simulink model "float_sch_PTSD"  (R2020a)
settings: Solver=VariableStepAuto  StartTime=0  StopTime=5  RelTol=1e-3
values from neighbouring files (symbols this model uses):
  buffer_rec = 30    [float_sch_run_PTSD.m]
  diff_th = [20:1.25:100]    [float_sch_run_PTSD.m]
  fs = 30000    [float_sch_run_LocalMaxima_AdaptiveThreshold.m]    (also in float_sch_run_LocalMaxima_HardThreshold.m; float_sch_run_PTSD.m; float_sch_run_Sample_AdaptiveThreshold.m; float_sch_run_Sample_HardThreshold.m)
  PLP = 22    [float_sch_run_PTSD.m]
  refractory = 10^-3    (= 0.001)    [float_sch_run_LocalMaxima_AdaptiveThreshold.m]    (also in float_sch_run_LocalMaxima_HardThreshold.m; float_sch_run_PTSD.m; float_sch_run_Sample_AdaptiveThreshold.m; float_sch_run_Sample_HardThreshold.m)
libraries: simulink x6, dsparch4 x2, dspstat3 x2, dspswit3 x1, hdlsllib x1
settings Model: Creator=sbuccelli  LastModifiedBy=diflo

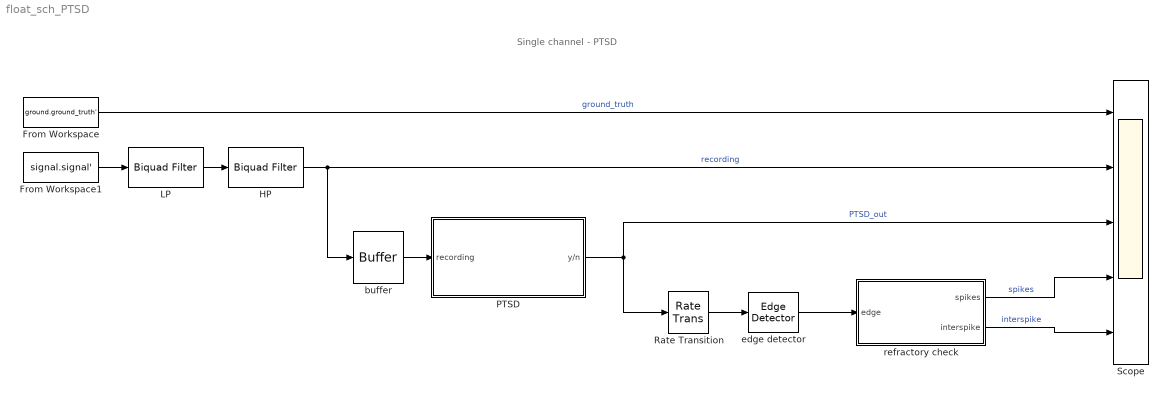
== system float_sch_PTSD ==
  note: Single channel - PTSD
  From Workspace : FromWorkspace  VariableName=ground.ground_truth'  SampleTime=1/fs
  From Workspace1 : FromWorkspace  VariableName=signal.signal'  SampleTime=1/fs
  HP : dsparch4/Biquad Filter  Tag=BlockMethodSubSystem  FilterSource=Dialog parameters  CoeffSource=Specify via dialog  FilterObject=BQF  IIRFiltStruct=Direct form II  BiQuadCoeffs=[1 -2 1 1 -1.93529438685999167 0.93912079880642374;1 -1 0 1 -0.939062505817492399 0]  ScaleValues=[0.968603796416603768;0.969531252908746199;1]  IC=0  ICnum=0  ICden=0  a0Flag=Warning  optimizeScaleValues=on  ScaleValueMode=Specify via input port (g)  roundingMode=Floor  overflowMode=off  scaleValueFracLength=14  denProdOutputFracLength=30  denAccumFracLength=30  secondMemoryFracLength=15
  LP : dsparch4/Biquad Filter  Tag=BlockMethodSubSystem  FilterSource=Dialog parameters  CoeffSource=Specify via dialog  FilterObject=BQF  IIRFiltStruct=Direct form II  BiQuadCoeffs=[1 1 0 1 -0.509525449494428795 0]  ScaleValues=[0.245237275252785547;1]  IC=0  ICnum=0  ICden=0  a0Flag=Warning  optimizeScaleValues=on  ScaleValueMode=Specify via input port (g)  roundingMode=Floor  overflowMode=off  scaleValueFracLength=14  denProdOutputFracLength=30  denAccumFracLength=30  secondMemoryFracLength=15
  PTSD : Subsystem
  Rate Transition : RateTransition  OutPortSampleTime=1/fs
  Scope : Scope  NumInputPorts=5
  buffer : Buffer  N=buffer_rec  V=buffer_overlap  OutputFrames=off
  edge detector : dspswit3/Edge Detector  InputProcessing=Columns as channels (frame based)
      settings: SourceProductBaseCode=DS
  refractory check : Subsystem
  wires:
  From Workspace/1 -> Scope/1  "ground_truth"
  buffer/1 -> PTSD/1(recording)
  From Workspace1/1 -> LP/1
  Rate Transition/1 -> edge detector/1
  PTSD/1(y/n) -> Scope/3, Rate Transition/1  "PTSD_out"
  refractory check/1(" spikes") -> Scope/4  "spikes"
  refractory check/2(interspike) -> Scope/5  "interspike"
  edge detector/1 -> refractory check/1(" edge  ")
  HP/1 -> Scope/2, buffer/1  "recording"
  LP/1 -> HP/1

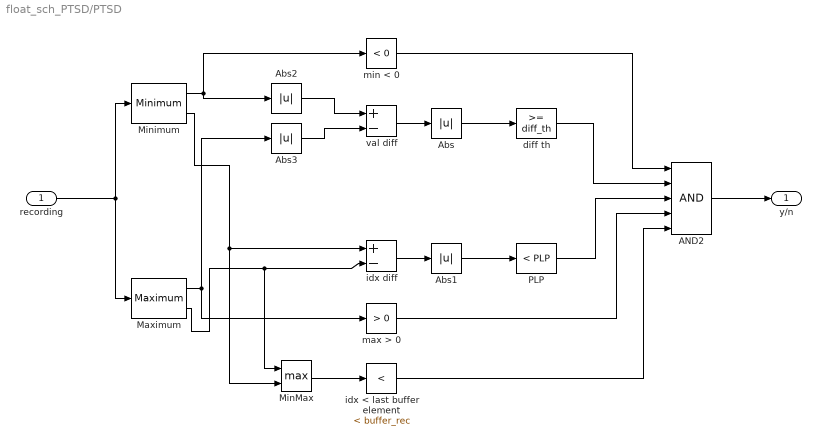
== system float_sch_PTSD/PTSD ==
  recording : Inport
  AND2 : Logic  Inputs=5  IconShape=distinctive  AllPortsSameDT=off  OutDataTypeStr=boolean
  Abs{,1..3} (4 alike) : Abs
  Maximum : dspstat3/Maximum  operation=maximum  fcn=Value and Index  indexBase=One  operateOver=Each column  Dimension=1  InputProcessing=Columns as channels (frame based)  reset=None  roiEnable=off  roiType=Rectangles  roiPortion=Entire ROI  roiOutput=Individual statistics for each ROI  roiFlag=off  roundingMode=Floor  overflowMode=off  accumDataTypeStr=Inherit: Same as product output  accumLastDataTypeStr=Inherit: Same as product output
  MinMax : MinMax  Function=max  Inputs=2
  Minimum : dspstat3/Minimum  operation=minimum  fcn=Value and Index  indexBase=One  operateOver=Each column  Dimension=1  InputProcessing=Columns as channels (frame based)  reset=None  roiEnable=off  roiType=Rectangles  roiPortion=Entire ROI  roiOutput=Individual statistics for each ROI  roiFlag=off  roundingMode=Floor  overflowMode=off
      settings: SourceProductBaseCode=DS
  PLP : simulink/Logic and Bit Operations/Compare To Constant  relop=<  const=PLP  OutDataTypeStr=boolean
  diff th : simulink/Logic and Bit Operations/Compare To Constant  relop=>=  const=diff_th  OutDataTypeStr=boolean
  idx < last buffer element : simulink/Logic and Bit Operations/Compare To Constant  relop=<  const=buffer_rec  OutDataTypeStr=boolean
  idx diff : Sum  Inputs=+-
  max > 0 : simulink/Logic and Bit Operations/Compare To Constant  relop=>  const=0  OutDataTypeStr=boolean
  min < 0 : simulink/Logic and Bit Operations/Compare To Constant  relop=<  const=0  OutDataTypeStr=boolean
  val diff : Sum  Inputs=+-
  y/n : Outport
  wires:
  Minimum/2 -> MinMax/2, idx diff/1
  Maximum/2 -> MinMax/1, idx diff/2
  val diff/1 -> Abs/1
  Maximum/1 -> Abs3/1, max > 0/1
  Abs1/1 -> PLP/1
  recording/1 -> Maximum/1, Minimum/1
  Abs/1 -> diff th/1
  idx diff/1 -> Abs1/1
  Minimum/1 -> Abs2/1, min < 0/1
  min < 0/1 -> AND2/1
  diff th/1 -> AND2/2
  AND2/1 -> y/n/1
  PLP/1 -> AND2/3
  max > 0/1 -> AND2/4
  Abs2/1 -> val diff/1
  Abs3/1 -> val diff/2
  MinMax/1 -> idx < last buffer element/1
  idx < last buffer element/1 -> AND2/5

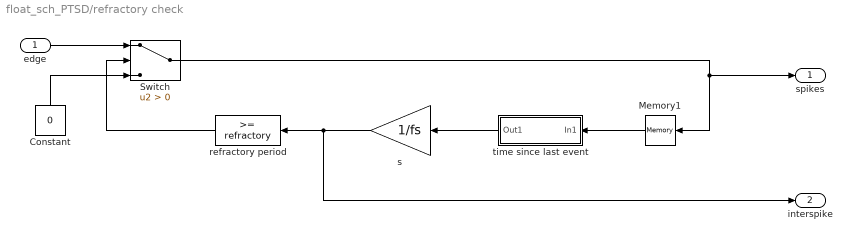
== system float_sch_PTSD/refractory check ==
  " edge  " : Inport
  Constant : Constant  Value=0
  Memory1 : Memory  InheritSampleTime=on
  Switch : Switch  Criteria=u2 > Threshold
  refractory period : simulink/Logic and Bit Operations/Compare To Constant  relop=>=  const=refractory  OutDataTypeStr=boolean
  s : Gain  Gain=1/fs  ParamDataTypeStr=double
  time since last event : Subsystem
  " spikes" : Outport
  interspike : Outport  Port=2
  wires:
  " edge  "/1 -> Switch/1
  Memory1/1 -> time since last event/1(In1)
  time since last event/1(Out1) -> s/1
  Constant/1 -> Switch/3
  s/1 -> refractory period/1, interspike/1
  Switch/1 -> " spikes"/1, Memory1/1
  refractory period/1 -> Switch/2

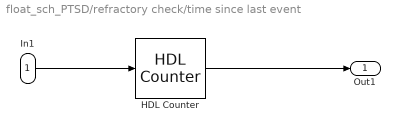
== system float_sch_PTSD/refractory check/time since last event ==
  In1 : Inport
  HDL Counter : hdlsllib/Sources/HDL Counter  CountType=Free running  CountInit=1  CountStep=1  CountMax=25  CountFromType=Initial value  CountFrom=1  CountResetPort=on  CountLoadPort=off  CountEnbPort=off  CountDirPort=off  CountDataType=Unsigned  CountWordLen=32  CountFracLen=0  CountSampTime=1
  Out1 : Outport
  wires:
  In1/1 -> HDL Counter/1
  HDL Counter/1 -> Out1/1
